simulink model "stateflow_FMU_test_shrd_lib"  (R2021b)
settings: Solver=FixedStepAuto  StartTime=0.0  StopTime=5.0  RelTol=1e-3
settings Model: Creator=lordx  LastModifiedBy=lordx
settings OptimizationCC: DefaultParameterBehavior=Inlined  EnhancedBackFolding=on  PassReuseOutputArgsAs=Individual arguments  ZeroExternalMemoryAtStartup=off  ZeroInternalMemoryAtStartup=off  OptimizeBlockOrder=speed  DifferentSizesBufferReuse=on  OptimizationCustomize=off  EfficientTunableParamExpr=on
settings DebuggingCC: ParameterTunabilityLossMsg=error
settings HardwareCC: TargetBitPerPointer=64  TargetBitPerSizeT=64  TargetBitPerPtrDiffT=64  TargetLongLongMode=on  TargetIntDivRoundTo=Zero  TargetEndianess=LittleEndian  TargetWordSize=64  TargetHWDeviceType=MATLAB Host  ProdEqTarget=off
settings SFSimCC: MATLABDynamicMemAlloc=off
settings RTWCC: Description=Embedded Coder (host-based shared library target)  SystemTargetFile=ert_shrlib.tlc  TemplateMakefile=ert_default_tmf  GenerateReport=on  RetainRTWFile=on  CodeExecutionProfiling=on  GenerateWebview=on  GenerateCodeMetricsReport=on
settings CodeAppCC: ForceParamTrailComments=on  IgnoreCustomStorageClasses=off  OperatorAnnotations=on  SimulinkDataObjDesc=on  SFDataObjDesc=on  InsertBlockDesc=on  StateflowObjectComments=on  MATLABSourceComments=on
settings STFCustomTargetCC: TargetLangStandard=C99 (ISO)  MultiwordLength=256  GenerateSampleERTMain=on  ParMdlRefBuildCompliant=on  CompOptLevelCompliant=on  CombineOutputUpdateFcns=on  ERTCustomFileBanners=on  SupportContinuousTime=off  SupportNonInlinedSFcns=off  RemoveResetFunc=on  MATLABClassNameForMDSCustomization=Simulink.SoftwareTarget.ERTCustomization  ModelStepFunctionPrototypeControlCompliant=on  GRTInterface=off  UseToolchainInfoCompliant=on  SystemTargetFile=ert_shrlib.tlc
settings ERTTargetCC: TargetLangStandard=C99 (ISO)  GenerateSampleERTMain=on  ConcurrentExecutionCompliant=off  CPPClassGenCompliant=off  InlinedParameterPlacement=NonHierarchical  RTWCAPISignals=on  RTWCAPIParams=on  RTWCAPIStates=on  RTWCAPIRootIO=on  ERTCustomFileTemplate=example_file_process.tlc  PreserveExpressionOrder=on  PreserveIfCondition=on

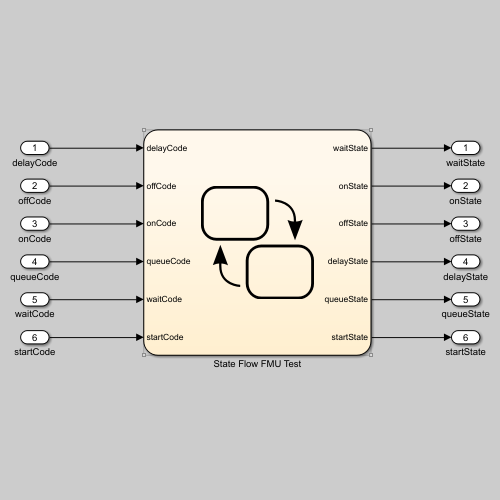
[thumbnail: Simulink's stored preview of the top-level diagram]
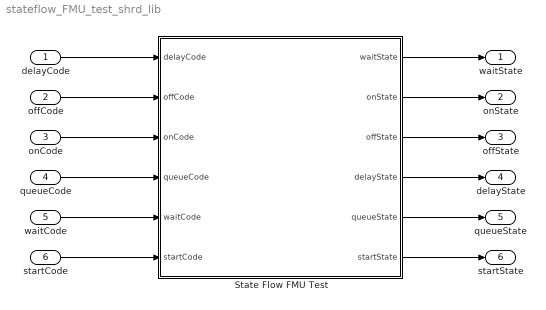
== system stateflow_FMU_test_shrd_lib ==
  delayCode : Inport
  offCode : Inport  Port=2
  onCode : Inport  Port=3
  queueCode : Inport  Port=4
  waitCode : Inport  Port=5
  startCode : Inport  Port=6
  State Flow FMU Test : Stateflow chart  TreatAsAtomicUnit=on
  waitState : Outport
  onState : Outport  Port=2
  offState : Outport  Port=3
  delayState : Outport  Port=4
  queueState : Outport  Port=5
  startState : Outport  Port=6
  wires:
  delayCode/1 -> State Flow FMU Test/1(delayCode)
  offCode/1 -> State Flow FMU Test/2(offCode)
  onCode/1 -> State Flow FMU Test/3(onCode)
  queueCode/1 -> State Flow FMU Test/4(queueCode)
  waitCode/1 -> State Flow FMU Test/5(waitCode)
  State Flow FMU Test/1(waitState) -> waitState/1
  State Flow FMU Test/2(onState) -> onState/1
  State Flow FMU Test/3(offState) -> offState/1
  State Flow FMU Test/4(delayState) -> delayState/1
  State Flow FMU Test/5(queueState) -> queueState/1
  startCode/1 -> State Flow FMU Test/6(startCode)
  State Flow FMU Test/6(startState) -> startState/1

== stateflow chart stateflow_FMU_test_shrd_lib/State Flow FMU Test ==
  state start/
    startState=1;
    delayState=1;
  state on/
    onState=1;
  state wait/
    waitState=1;
  state delay/
    delayState==1;
  state queue/
    queueState==1;
  state off/
    offState==1;
  (default) -> start
  off -> start [order 1] : [startCode==0 && offCode==0]
  start -> off [order 2] : [offCode==1 && startCode==0]
  start -> on [order 1] : [startCode==1 && onCode==1]
  off -> on [order 2] : [onCode==1]
  on -> off [order 2] : [offCode==1]
  on -> wait [order 1] : [waitCode==1 && onCode == 1]
  wait -> on [order 1] : [waitCode==1 && onCode == 0]
  wait -> delay [order 2] : [delayCode==1]
  delay -> wait [order 1] : [delayCode==0]
  delay -> queue [order 2] : [queueCode==1]
  queue -> delay [order 1] : [queueCode==1]
  queue -> off [order 2] : [offCode==1]
  data: waitState output double; onState output double; offState output double; delayState output double; delayCode input; offCode input; onCode input; queueCode input; queueState output double; waitCode input; startCode input double; startState output double
